simulink model "fuzzy_pi_simulink"  (R2020a)
settings: Solver=ode23tb  StartTime=0.0  StopTime=100  RelTol=1e-3  EnableMultiTasking=on
values from neighbouring files (symbols this model uses):
  fuzzy_K0 = pid_Kp / pid_Ti    (= 0.555191661948)    [fuzzy_pid.m]
  fuzzy_K1 = fuzzy_K0 * alpha_beta(1)    [fuzzy_pid.m]
  fuzzy_Kd = alpha_beta(1) * fuzzy_Ke    [fuzzy_pid.m]
  fuzzy_Ke = 1    [fuzzy_pid.m]
  pid_Kd = Tcr / 8    (= 0.8)    [fuzzy_pid.m]
  pid_Ki = 2 / Tcr    (= 0.3125)    [fuzzy_pid.m]
  pid_Kp = 0.6 * Kcr    (= 1.77661331824)    [fuzzy_pid.m]
libraries: fuzblock x1, simulink x1
settings Model: Creator=paulo.costa  LastModifiedBy=paulo
settings DataIOCC: LimitDataPoints=on  SaveFormat=Array  ReturnWorkspaceOutputs=off
settings OptimizationCC: LifeSpan=inf
settings DebuggingCC: UnderspecifiedInitializationDetection=Classic  MergeDetectMultiDrivingBlocksExec=none  SolverPrmCheckMsg=warning  StateNameClashWarn=warning  SFUnexpectedBacktrackingDiag=warning  SFNoUnconditionalDefaultTransitionDiag=warning  SFExecutionAtInitializationDiag=none  ArithmeticOperatorsInVariantConditions=warning
settings HardwareCC: ProdBitPerPointer=32  ProdBitPerSizeT=32  ProdBitPerPtrDiffT=32  ProdLargestAtomicFloat=None  ProdIntDivRoundTo=Undefined  ProdEndianess=Unspecified  ProdWordSize=32  ProdHWDeviceType=32-bit Generic
settings ModelReferenceCC: PropagateSignalLabelsOutOfModel=off
settings SFSimCC: SimUseLocalCustomCode=off  CustomCodeUndefinedFunction=UseInterfaceOnly
settings RTWCC: RTWUseLocalCustomCode=off
settings CodeAppCC: StateflowObjectComments=on
settings GRTTargetCC: TargetLangStandard=C89/C90 (ANSI)
settings ConfigComp: CovMetricSettings=dw  CovHtmlReporting=on  CovSaveCumulativeToWorkspaceVar=on  CovSaveSingleToWorkspaceVar=on  CovExternalEMLEnable=off

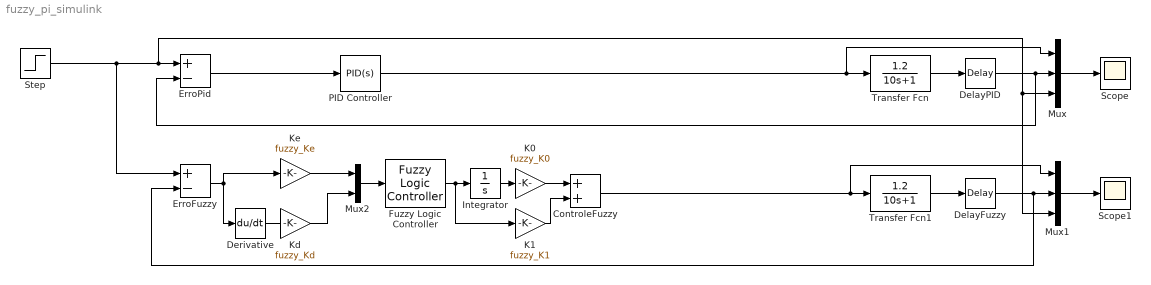
== system fuzzy_pi_simulink ==
  ControleFuzzy : Sum
  DelayFuzzy : TransportDelay  DelayTime=2
  DelayPID : TransportDelay  DelayTime=2
  Derivative : Derivative
  ErroFuzzy : Sum  Inputs=+-
  ErroPid : Sum  Inputs=+-
  Fuzzy Logic Controller : fuzblock/Fuzzy Logic  Controller  FIS=fuzzy_pi  OutputSampleNumber=101  DataType=double  FuzzifiedInputs=off  RuleFiringStrengths=off  RuleOutputs=off  AggregatedOutputs=off  SimulateUsing=Interpreted execution  OutOfRangeInputValueMessage=warning  NoRuleFiredMessage=warning  EmptyOutputFuzzySetMessage=warning
  Integrator : Integrator
  K0 : Gain  Gain=fuzzy_K0
  K1 : Gain  Gain=fuzzy_K1
  Kd : Gain  Gain=fuzzy_Kd
  Ke : Gain  Gain=fuzzy_Ke
  Mux : Mux  Inputs=3
  Mux1 : Mux  Inputs=3
  Mux2 : Mux  Inputs=2
  PID Controller : simulink/Continuous/PID Controller  Controller=PID  Form=Parallel  TimeDomain=Continuous-time  UseExternalTs=off  SampleTime=1  IntegratorMethod=Forward Euler  FilterMethod=Forward Euler  ControllerParametersSource=internal  P=pid_Kp  I=pid_Ki  D=pid_Kd  UseFilter=on  N=100  TunerSelectOption=Transfer Function Based (PID Tuner App)  InitialConditionSource=internal  InitialConditionForIntegrator=0  InitialConditionForFilter=0  DifferentiatorICPrevScaledInput=0  ExternalReset=none  TrackingMode=off  Kt=1  LimitOutput=off  UpperSaturationLimit=inf  LowerSaturationLimit=-inf  LinearizeAsGain=on  AntiWindupMode=none  Kb=1  POutMin=[]  POutMax=[]  IOutMin=[]  IOutMax=[]  DOutMin=[]  DOutMax=[]  NOutMin=[]  NOutMax=[]  SumOutMin=[]  SumOutMax=[]  SaturationOutMin=[]  SaturationOutMax=[]  PParamMin=[]  PParamMax=[]  IParamMin=[]  IParamMax=[]  DParamMin=[]  DParamMax=[]  NParamMin=[]  NParamMax=[]  KbParamMin=[]  KbParamMax=[]  KtParamMin=[]  KtParamMax=[]  KbOutMin=[]  KbOutMax=[]  KtOutMin=[]  KtOutMax=[]  IntegratorOutMin=[]  IntegratorOutMax=[]  FilterOutMin=[]  FilterOutMax=[]  SumI1OutMin=[]  SumI1OutMax=[]  SumI2OutMin=[]  SumI2OutMax=[]  SumI3OutMin=[]  SumI3OutMax=[]  SumI4OutMin=[]  SumI4OutMax=[]  SumDOutMin=[]  SumDOutMax=[]  DifferentiatorOutMin=[]  DifferentiatorOutMax=[]  FilterDiffOutCoefMin=[]  FilterDiffOutCoefMax=[]  ReciprocalOutMin=[]  ReciprocalOutMax=[]  SumDenOutMin=[]  SumDenOutMax=[]  SumNumOutMin=[]  SumNumOutMax=[]  DivideOutMin=[]  DivideOutMax=[]  UdiffTsProdOutMin=[]  UdiffTsProdOutMax=[]  NTsProdOutMin=[]  NTsProdOutMax=[]  UintegralTsProdOutMin=[]  UintegralTsProdOutMax=[]  UngainTsProdOutMin=[]  UngainTsProdOutMax=[]  IntegratorContinuousStateAttributes=''  IntegratorStateMustResolveToSignalObject=off  IntegratorRTWStateStorageClass=Auto  FilterContinuousStateAttributes=''  FilterStateMustResolveToSignalObject=off  FilterRTWStateStorageClass=Auto  ParallelPVariant=InternalParameters  IdealPVariant=Disabled  IVariant=InternalParameters  DVariant=InternalParameters  IntegratorVariant=Continuous  SatVariant=Disabled  AWVariant=Passthrough  PCopyVariant=Disabled  TRVariant=Disabled  FdbkBlocksVariant=Forward  IdealPFdbkVariant=Disabled  SatFdbkVariant=Disabled  DerivativeFilterVariant=ContFilter  NVariant=InternalParameters  NCopyVariant=Disabled  FilterICVariant=InternalICsFilter  IntegratorICVariant=InternalICs  ExternalResetVariant=Disabled  TRSumVariant=Passthrough  SumFdbkVariant=Disabled  SumVariant=Sum_PID  TsampFilterVariant=InternalTs  TsampNgainVariant=Passthrough  TsampIntegralVariant=Passthrough
  Scope : Scope
  Scope1 : Scope
  Step : Step  SampleTime=0
  Transfer Fcn : TransferFcn  Numerator=[1.2]  Denominator=[10 1]
  Transfer Fcn1 : TransferFcn  Numerator=[1.2]  Denominator=[10 1]
  wires:
  Mux/1 -> Scope/1
  DelayFuzzy/1 -> ErroFuzzy/2, Mux1/2
  Mux1/1 -> Scope1/1
  Fuzzy Logic Controller/1 -> K1/1, Integrator/1
  ErroFuzzy/1 -> Derivative/1, Ke/1
  Mux2/1 -> Fuzzy Logic Controller/1
  Derivative/1 -> Mux2/2
  DelayPID/1 -> ErroPid/2, Mux/2
  ErroPid/1 -> PID Controller/1
  Step/1 -> Mux/3, Mux1/3, ErroPid/1, ErroFuzzy/1
  PID Controller/1 -> Transfer Fcn/1, Mux/1
  K0/1 -> ControleFuzzy/1
  K1/1 -> ControleFuzzy/2
  ControleFuzzy/1 -> Transfer Fcn1/1, Mux1/1
  Integrator/1 -> K0/1
  Ke/1 -> Mux2/1
  Transfer Fcn/1 -> DelayPID/1
  Transfer Fcn1/1 -> DelayFuzzy/1
